simulink model "AR_HeadLampSWC"  (Simulink 8.0)
settings: Solver=FixedStepDiscrete  SolverMode=SingleTasking  StartTime=0.0  StopTime=inf  FixedStep=0.01  RelTol=1e-3
model workspace (MAT data in the model file):
  SLAMConfig__ATPP : SLAM.Root (value not decoded)
  SLAMConfig_47_ATPP : SLAM.Root (value not decoded)
CloseFcn:
  | rtwprivate ssgencode ModelCloseRequest testAutosar
settings Model: Creator=Shucheng  LastModifiedBy=sdong
settings DataIOCC: LimitDataPoints=off  SaveFormat=StructureWithTime  SignalLoggingSaveFormat=ModelDataLogs
settings OptimizationCC: InlineParams=on  ZeroExternalMemoryAtStartup=off  ZeroInternalMemoryAtStartup=off  OptimizeModelRefInitCode=on  LifeSpan=1
settings DebuggingCC: FcnCallInpInsideContextMsg=UseLocalSettings  StrictBusMsg=Warning
settings HardwareCC: TargetHWDeviceType=32-bit Generic
settings RTWCC: SystemTargetFile=autosar.tlc  GenCodeOnly=on  TemplateMakefile=ert_default_tmf  Description=AUTOSAR  GenerateReport=on  ProcessScript=autosar_make_rtw_hook  IncludeHyperlinkInReport=on  LaunchReport=on  GenerateCodeInfo=on
settings CodeAppCC: GenerateComments=off  IgnoreCustomStorageClasses=off  MaxIdLength=120  SimulinkBlockComments=off
settings STFCustomTargetCC: CodeReplacementLibrary=ANSI_C  ParMdlRefBuildCompliant=on  CompOptLevelCompliant=on  IncludeMdlTerminateFcn=off  CombineOutputUpdateFcns=on  SuppressErrorStatus=on  ERTFirstTimeCompliant=on  ERTCustomFileBanners=on  SupportAbsoluteTime=off  MultiInstanceERTCode=on  SupportNonFinite=off  SupportComplex=off  SupportContinuousTime=off  SupportNonInlinedSFcns=off  AutosarCompliant=on  GRTInterface=off  SystemTargetFile=autosar.tlc
settings ERTTargetCC: CodeReplacementLibrary=ANSI_C  MultiwordLength=2048  ConcurrentExecutionCompliant=off  IncludeMdlTerminateFcn=off  SuppressErrorStatus=on  SupportAbsoluteTime=off  MultiInstanceERTCode=on  SupportNonFinite=off  SupportComplex=off  ModelStepFunctionPrototypeControlCompliant=off  CPPClassGenCompliant=off  AutosarCompliant=on  ExtModeMexFile=noextcomm  InlinedParameterPlacement=NonHierarchical  ERTCustomFileTemplate=example_file_process.tlc  ERTFilePackagingFormat=Compact  ConvertIfToSwitch=off  SuppressUnreachableDefaultCases=off
settings CustomProperty: DataType=RTWOptions_EnumType__toolbox_rtw_targets_autosar_autosar_autosar_1_2AutosarSchemaVersion  Value=3.0
settings EnumStrPairs: String=2.1

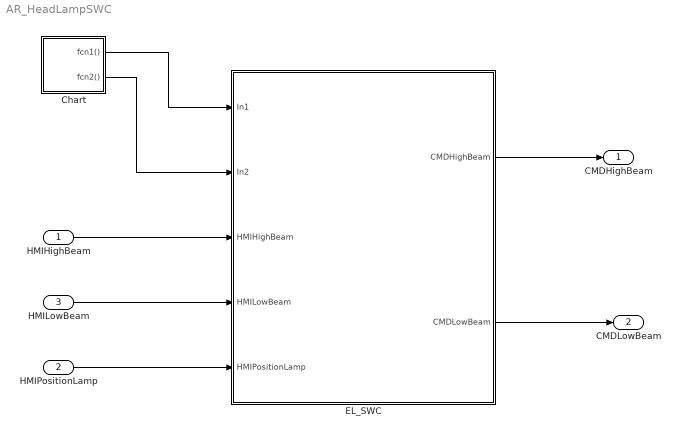
== system AR_HeadLampSWC ==
  HMIHighBeam : Inport
  HMIPositionLamp : Inport  Port=2
  HMILowBeam : Inport  Port=3
  Chart : Stateflow chart  TreatAsAtomicUnit=on
  EL_SWC : Subsystem
  CMDHighBeam : Outport
  CMDLowBeam : Outport  Port=2
  wires:
  HMIHighBeam/1 -> EL_SWC/3(HMIHighBeam)
  HMILowBeam/1 -> EL_SWC/4(HMILowBeam)
  HMIPositionLamp/1 -> EL_SWC/5(HMIPositionLamp)
  EL_SWC/1(CMDHighBeam) -> CMDHighBeam/1
  EL_SWC/2(CMDLowBeam) -> CMDLowBeam/1
  Chart/1(fcn1()) -> EL_SWC/1(In1)
  Chart/2(fcn2()) -> EL_SWC/2(In2)

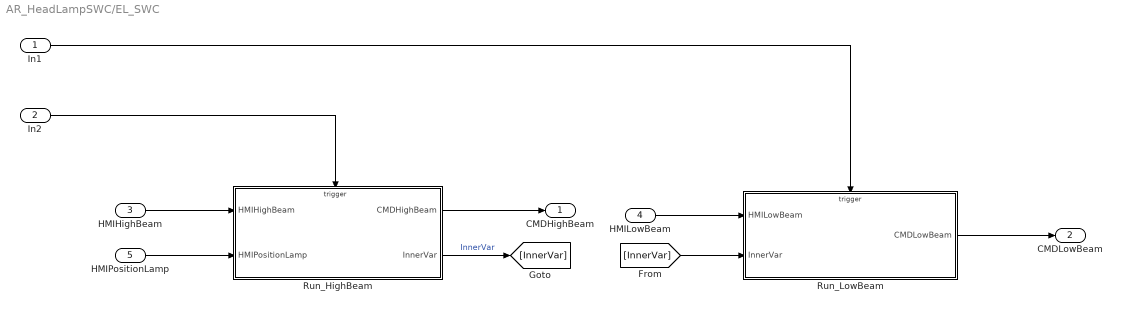
== system AR_HeadLampSWC/EL_SWC ==
  In1 : Inport
  In2 : Inport  Port=2
  HMIHighBeam : Inport  Port=3
  HMILowBeam : Inport  Port=4
  HMIPositionLamp : Inport  Port=5
  Run_HighBeam : Subsystem  TreatAsAtomicUnit=on
  Run_LowBeam : Subsystem  TreatAsAtomicUnit=on
  CMDHighBeam : Outport
  CMDLowBeam : Outport  Port=2
  wires:
  HMIHighBeam/1 -> Run_HighBeam/1(HMIHighBeam)
  Run_HighBeam/1(CMDHighBeam) -> CMDHighBeam/1
  HMIPositionLamp/1 -> Run_HighBeam/2(HMIPositionLamp)
  HMILowBeam/1 -> Run_LowBeam/1(HMILowBeam)
  Run_LowBeam/1(CMDLowBeam) -> CMDLowBeam/1
  Run_HighBeam/2(InnerVar) -> [InnerVar]  "InnerVar"
  [InnerVar] -> Run_LowBeam/2(InnerVar)
  In1/1 -> Run_LowBeam/Trigger
  In2/1 -> Run_HighBeam/Trigger

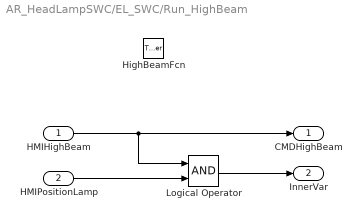
== system AR_HeadLampSWC/EL_SWC/Run_HighBeam ==
  HMIHighBeam : Inport
  HMIPositionLamp : Inport  Port=2
  HighBeamFcn : TriggerPort  TriggerType=function-call
  Logical Operator : Logic  AllPortsSameDT=off  OutDataTypeStr=boolean
  CMDHighBeam : Outport
  InnerVar : Outport  Port=2
  wires:
  HMIHighBeam/1 -> CMDHighBeam/1, Logical Operator/1
  HMIPositionLamp/1 -> Logical Operator/2
  Logical Operator/1 -> InnerVar/1

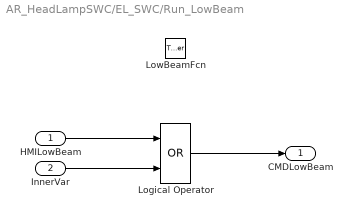
== system AR_HeadLampSWC/EL_SWC/Run_LowBeam ==
  HMILowBeam : Inport
  InnerVar : Inport  Port=2
  LowBeamFcn : TriggerPort  TriggerType=function-call
  Logical Operator : Logic  Operator=OR  AllPortsSameDT=off  OutDataTypeStr=boolean
  CMDLowBeam : Outport
  wires:
  HMILowBeam/1 -> Logical Operator/1
  InnerVar/1 -> Logical Operator/2
  Logical Operator/1 -> CMDLowBeam/1

== stateflow chart Chart ==
  (default) -> (junction 5)
  (junction 5) -> (junction 6) : {
      | fcn1;
      | fcn2;
      | }
  events: fcn1 output FUNCTION_CALL_EVENT; fcn2 output FUNCTION_CALL_EVENT
